simulink subsystem "Visualization_shared_subsystem"  (R2022b)
settings: Solver=VariableStepAuto  StartTime=0.0  StopTime=10.0  RelTol=1e-3
undefined symbols (not defined in the file): coord_xaxis_len, coord_yaxis_len, coord_zaxis_len, X, Y, Z
libraries: sm_lib x110, nesl_utility x21
(part 3 of 3)

== matlab function Visualization_shared_subsystem/xdof_switch ==
  data: q input; q_7dof output; q_p input; q_pp input; q_p_7dof output; q_pp_7dof output; param_robot parameter
function [q_7dof, q_p_7dof, q_pp_7dof] = fcn(q, q_p, q_pp, param_robot)
% In 7dof case q_7dof = q, q_p_7dof = q_p and q_pp_7dof = q_pp
% In 6dof case only the nonfixed joints are changed.

q_0_ref    = param_robot.q_0_ref; % 7DOF q_0_init
q_0_p_ref  = param_robot.q_0_p_ref; % 7DOF q_0_init
q_0_pp_ref = param_robot.q_0_pp_ref; % 7DOF q_0_init

% Overwrite non fixed joint angles
q_0_ref(param_robot.n_indices)    = q;
q_0_p_ref(param_robot.n_indices)  = q_p;
q_0_pp_ref(param_robot.n_indices) = q_pp;

q_7dof    = q_0_ref;
q_p_7dof  = q_0_p_ref;
q_pp_7dof = q_0_pp_ref;

== matlab function Visualization_shared_subsystem/show pritzi force arrows/MATLAB Function1 ==
  data: q input; px output; py output; pz output; f_ext input; param_robot parameter
function [px, py, pz] = fcn(q, f_ext, param_robot)
    %J=geo_jacobian_endeffector(q,param_robot);
    H=hom_transform_endeffector(q,param_robot);

    if norm(f_ext) < 1e-3
        px = 0;
        py = 0;
        pz = 0;
    else
        p = H(1:3, 4);
        px = p(1);
        py = p(2);
        pz = p(3);
    end
end

== matlab function Visualization_shared_subsystem/show pritzi force arrows/MATLAB Function2 ==
  data: q input; px output; py output; pz output; f_ext input; param_robot parameter
function [px, py, pz] = fcn(q, f_ext, param_robot)
    %J=geo_jacobian_endeffector(q,param_robot);
    H=hom_transform_endeffector(q,param_robot);

    if norm(f_ext) < 1e-3
        px = 0;
        py = 0;
        pz = 0;
    else
        p = H(1:3, 4);
        px = p(1);
        py = p(2);
        pz = p(3);
    end
end

== matlab function Visualization_shared_subsystem/show pritzi force arrows/calc_rotations ==
  data: fx input; Rx output; Ry output; Rz output; fy input; fz input
function [Rx, Ry, Rz] = fcn(fx, fy, fz)
    Rx = -atan2(fy, fz);
    Ry = atan2(fx, sqrt(fy^2 + fz^2));
    Rz = 0;
end

== matlab function Visualization_shared_subsystem/show pritzi force arrows/calc_rotations1 ==
  data: taux input; Rx output; Ry output; Rz output; tauy input; tauz input
function [Rx, Ry, Rz] = fcn(taux, tauy, tauz)
    Rx = -atan2(tauy, tauz);
    Ry = atan2(taux, sqrt(tauy^2 + tauz^2));
    Rz = 0;
end
